simulink model "my_quad"  (Simulink 7.3)
settings: Solver=ode45  StartTime=0.0  StopTime=50  RelTol=1e-3
settings Model: Creator=The MathWorks Inc.  LastModifiedBy=sn00632  ExtModeTrigMode=oneshot  ExtModeArmWhenConnect=off  ExtModeAutoUpdateStatusClock=off
settings DataIOCC: LimitDataPoints=off  SaveFormat=StructureWithTime  SaveState=on  OutputSaveName=yout1
settings OptimizationCC: BlockReduction=off  BooleanDataType=off  InlineInvariantSignals=on  InitFltsAndDblsToZero=on
settings DebuggingCC: SaveWithParameterizedLinksMsg=none  SignalResolutionControl=TryResolveAllWithWarning  SolverPrmCheckMsg=none  MultiTaskDSMMsg=warning  MultiTaskCondExecSysMsg=none  StrictBusMsg=None
settings HardwareCC: TargetUnknown=on
settings RTWCC: IncludeERTFirstTime=on
settings GRTTargetCC: TargetFcnLib=ansi_tfl_tmw.mat

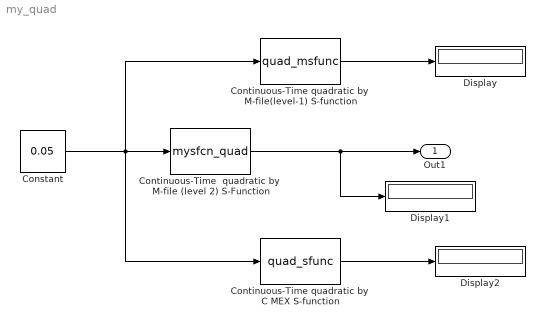
== system my_quad ==
  Constant : Constant  Value=0.05  OutDataType=sfix(16)  OutScaling=2^0
  Continuous-Time quadratic by  C MEX S-function : S-Function  FunctionName=quad_sfunc  EnableBusSupport=off
      mask Display: disp('y=ax^2+bx+c')
  Continuous-Time quadratic by  M-file(level-1) S-function : S-Function  FunctionName=quad_msfunc  Parameters=3,2,1  EnableBusSupport=off
      mask Display: disp('y=ax^2+bx+c')
  Continuous-Time  quadratic by  M-file (level 2) S-Function : M-S-Function  FunctionName=mysfcn_quad  Parameters=3,2,1  mask(S-Function: quad_sfunc){a=3, b=2, c=1}
      mask prompts: a "Input coefficient a:"; b "Input coefficient b:"; c "Input coefficient c:"
      mask help: This is a S-Funciton block which calculates a quadratic value.
      mask Display: disp('y=ax^2+bx+c')
  Display : Display
  Display1 : Display
  Display2 : Display
  Out1 : Outport  OutDataType=sfix(16)  OutScaling=2^0  InitialOutput=0
  wires:
  Constant/1 -> Continuous-Time  quadratic by  M-file (level 2) S-Function/1, Continuous-Time quadratic by  M-file(level-1) S-function/1, Continuous-Time quadratic by  C MEX S-function/1
  Continuous-Time  quadratic by  M-file (level 2) S-Function/1 -> Out1/1, Display1/1
  Continuous-Time quadratic by  M-file(level-1) S-function/1 -> Display/1
  Continuous-Time quadratic by  C MEX S-function/1 -> Display2/1
